simulink model "taller5_bloques_PID"  (R2020a)
settings: Solver=FixedStepAuto  StartTime=0.0  StopTime=.25  FixedStep=0.0001  RelTol=1e-3
values from neighbouring files (symbols this model uses):
  den = [1 R/L 1/(L*Cap)]    [taller5.m]
  num = 1/(L*Cap)    (= 45454.5454545)    [taller5.m]
settings Model: Creator=Personal  LastModifiedBy=Personal
settings SolverCC: ZeroCrossAlgorithm=Adaptive
settings DebuggingCC: IgnoredZcDiagnostic=none

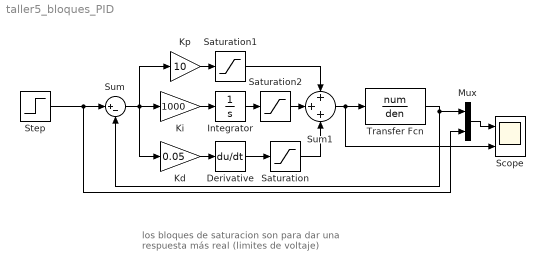
== system taller5_bloques_PID ==
  note: los bloques de saturacion son para
      | dar una respuesta más real (limites de voltaje)
  Derivative : Derivative
  Integrator : Integrator
  Kd : Gain  Gain=0.05
  Ki : Gain  Gain=1000
  Kp : Gain  Gain=10
  Mux : Mux  Inputs=2
  Saturation : Saturate  UpperLimit=15  LowerLimit=-15
  Saturation1 : Saturate  UpperLimit=15  LowerLimit=-15
  Saturation2 : Saturate  UpperLimit=15  LowerLimit=-15
  Scope : Scope  NumInputPorts=2
  Step : Step  Time=0.01  After=5  SampleTime=0
  Sum : Sum  Inputs=|+-
  Sum1 : Sum  Inputs=+++
  Transfer Fcn : TransferFcn  Numerator=num  Denominator=den
  wires:
  Transfer Fcn/1 -> Mux/1, Sum/2
  Sum/1 -> Kp/1, Kd/1, Ki/1
  Sum1/1 -> Scope/2, Transfer Fcn/1
  Ki/1 -> Integrator/1
  Kd/1 -> Derivative/1
  Derivative/1 -> Saturation/1
  Kp/1 -> Saturation1/1
  Integrator/1 -> Saturation2/1
  Saturation2/1 -> Sum1/2
  Saturation1/1 -> Sum1/1
  Mux/1 -> Scope/1
  Step/1 -> Mux/2, Sum/1
  Saturation/1 -> Sum1/3
